simulink model "cv6_sim"  (R2023b)
settings: Solver=VariableStepAuto  StartTime=0.0  StopTime=10.0  RelTol=1e-6  AbsTol=1e-6
settings Model: Creator=Lenovo  LastModifiedBy=miroh
settings OptimizationCC: ReuseModelBlockBuffer=off

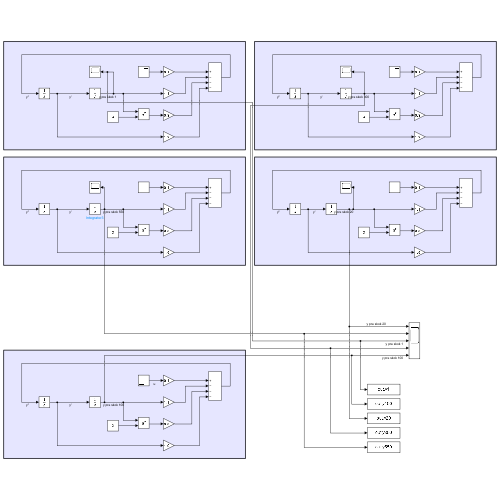
[thumbnail: Simulink's stored preview of the top-level diagram]
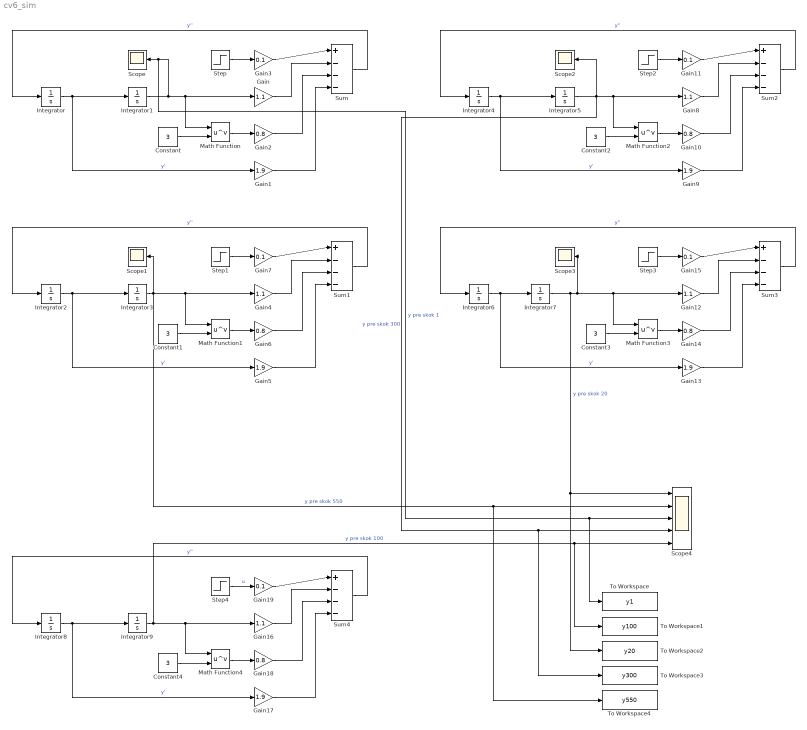
== system cv6_sim ==
  Constant{,1..4} (5 alike) : Constant  Value=3
  Gain{,4,8,12,16} (5 alike) : Gain  Gain=1.1
  Gain{1,5,9,13,17} (5 alike) : Gain  Gain=1.9
  Gain{2,6,10,14,18} (5 alike) : Gain  Gain=0.8
  Gain{3,7,11,15,19} (5 alike) : Gain  Gain=0.1
  Integrator{,1..9} (10 alike) : Integrator
  Math Function{,1..4} (5 alike) : Math  Operator=pow
  Scope{,1..3} (4 alike) : Scope
  Scope4 : Scope  NumInputPorts=5
  Step : Step  SampleTime=0
  Step1 : Step  Time=0  After=550  SampleTime=0
  Step2 : Step  Time=0  After=300  SampleTime=0
  Step3 : Step  After=20  SampleTime=0
  Step4 : Step  Time=0  After=100  SampleTime=0
  Sum{,1..4} (5 alike) : Sum  Inputs=|+---
  To Workspace : ToWorkspace  VariableName=y1  SaveFormat=Timeseries  SampleTime=-1
  To Workspace1 : ToWorkspace  VariableName=y100  SaveFormat=Timeseries  SampleTime=-1
  To Workspace2 : ToWorkspace  VariableName=y20  SaveFormat=Timeseries  SampleTime=-1
  To Workspace3 : ToWorkspace  VariableName=y300  SaveFormat=Timeseries  SampleTime=-1
  To Workspace4 : ToWorkspace  VariableName=y550  SaveFormat=Timeseries  SampleTime=-1
  wires:
  Integrator/1 -> Gain1/1, Integrator1/1  "y'"
  Integrator1/1 -> Scope4/3, To Workspace/1, Scope/1, Math Function/1, Gain/1  "y pre skok 1"
  Sum/1 -> Integrator/1  "y''"
  Constant/1 -> Math Function/2
  Math Function/1 -> Gain2/1
  Step/1 -> Gain3/1
  Gain3/1 -> Sum/1
  Gain/1 -> Sum/2
  Gain2/1 -> Sum/3
  Gain1/1 -> Sum/4
  Gain5/1 -> Sum1/4
  Constant1/1 -> Math Function1/2
  Gain7/1 -> Sum1/1
  Step1/1 -> Gain7/1
  Gain6/1 -> Sum1/3
  Integrator3/1 -> Gain4/1, Math Function1/1, To Workspace4/1, Scope4/2, Scope1/1  "y pre skok 550"
  Sum1/1 -> Integrator2/1  "y''"
  Math Function1/1 -> Gain6/1
  Gain4/1 -> Sum1/2
  Integrator2/1 -> Gain5/1, Integrator3/1  "y'"
  Gain9/1 -> Sum2/4
  Constant2/1 -> Math Function2/2
  Gain11/1 -> Sum2/1
  Step2/1 -> Gain11/1
  Gain10/1 -> Sum2/3
  Integrator5/1 -> To Workspace3/1, Scope4/4, Scope2/1, Math Function2/1, Gain8/1  "y pre skok 300"
  Sum2/1 -> Integrator4/1  "y''"
  Math Function2/1 -> Gain10/1
  Gain8/1 -> Sum2/2
  Integrator4/1 -> Gain9/1, Integrator5/1  "y'"
  Gain13/1 -> Sum3/4
  Constant3/1 -> Math Function3/2
  Gain15/1 -> Sum3/1
  Step3/1 -> Gain15/1
  Gain14/1 -> Sum3/3
  Integrator7/1 -> Scope3/1, Math Function3/1, Gain12/1, To Workspace2/1, Scope4/1  "y pre skok 20"
  Sum3/1 -> Integrator6/1  "y''"
  Math Function3/1 -> Gain14/1
  Gain12/1 -> Sum3/2
  Integrator6/1 -> Gain13/1, Integrator7/1  "y'"
  Integrator8/1 -> Gain17/1, Integrator9/1  "y'"
  Gain18/1 -> Sum4/3
  Math Function4/1 -> Gain18/1
  Gain16/1 -> Sum4/2
  Sum4/1 -> Integrator8/1  "y''"
  Integrator9/1 -> Scope4/5, To Workspace1/1, Gain16/1, Math Function4/1  "y pre skok 100"
  Step4/1 -> Gain19/1  "u"
  Gain19/1 -> Sum4/1
  Gain17/1 -> Sum4/4
  Constant4/1 -> Math Function4/2
